simulink library "driver_model_lib"  (R2022b)
settings: Solver=VariableStepAuto  StartTime=0.0  StopTime=10.0  RelTol=1e-3
settings Model: Creator=dr_pa  LastModifiedBy=dr_pa

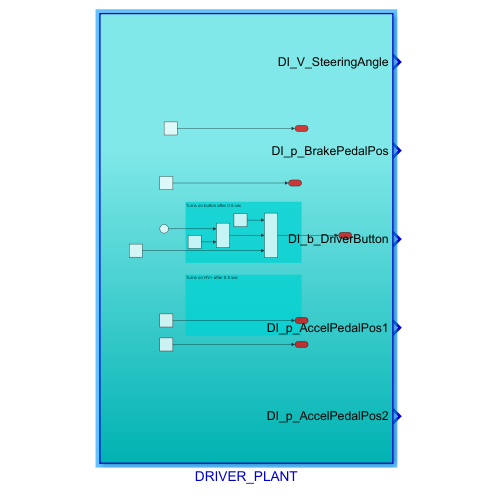
[thumbnail: Simulink's stored preview of the top-level diagram]
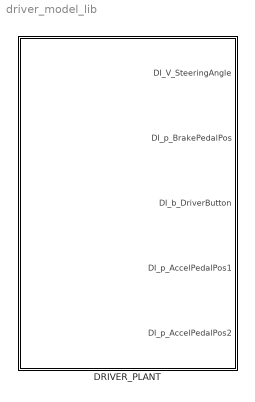
== system driver_model_lib ==
  DRIVER_PLANT : Subsystem

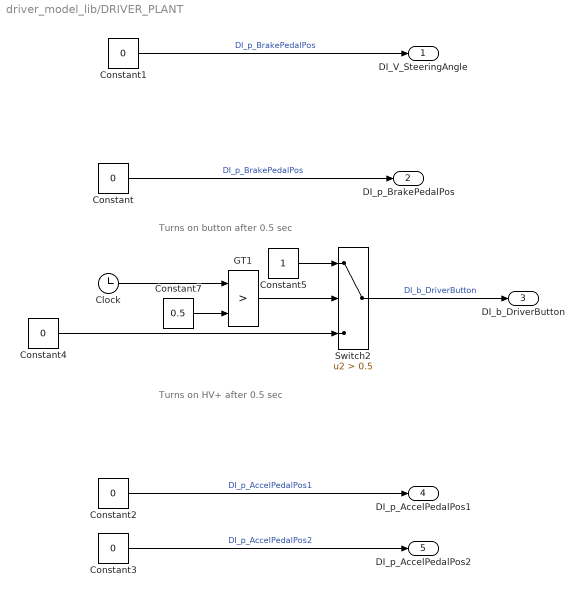
== system driver_model_lib/DRIVER_PLANT ==
  note: Turns on HV+ after 0.5 sec
  note: Turns on button after 0.5 sec
  Clock : Clock
  Constant{,1..4} (5 alike) : Constant  Value=0
  Constant5 : Constant
  Constant7 : Constant  Value=0.5
  GT1 : RelationalOperator  Operator=>  OutDataTypeStr=boolean  RndMeth=Simplest  InputSameDT=off
  Switch2 : Switch  Criteria=u2 > Threshold  Threshold=0.5  OutDataTypeStr=uint8  SaturateOnIntegerOverflow=off  InputSameDT=off
  DI_V_SteeringAngle : Outport
  DI_p_BrakePedalPos : Outport  Port=2
  DI_b_DriverButton : Outport  Port=3
  DI_p_AccelPedalPos1 : Outport  Port=4
  DI_p_AccelPedalPos2 : Outport  Port=5
  wires:
  Constant/1 -> DI_p_BrakePedalPos/1  "DI_p_BrakePedalPos"
  Switch2/1 -> DI_b_DriverButton/1  "DI_b_DriverButton"
  Constant3/1 -> DI_p_AccelPedalPos2/1  "DI_p_AccelPedalPos2"
  Constant2/1 -> DI_p_AccelPedalPos1/1  "DI_p_AccelPedalPos1"
  Clock/1 -> GT1/1
  Constant5/1 -> Switch2/1
  Constant4/1 -> Switch2/3
  Constant7/1 -> GT1/2
  GT1/1 -> Switch2/2
  Constant1/1 -> DI_V_SteeringAngle/1  "DI_p_BrakePedalPos"
